simulink model "compare"  (R2024b)
settings: Solver=FixedStepAuto  StartTime=0.0  StopTime=200  FixedStep=1/fs  RelTol=1e-3
values from neighbouring files (symbols this model uses):
  s = 1i * omega_full    [find_best_kc.m]
libraries: simulink_extras x4, dspfdesign x2, slctrl_linear x1, cstblocks x1, slctrl_fre x1
settings Model: Creator=caohuaqi  LastModifiedBy=Caohuaqi

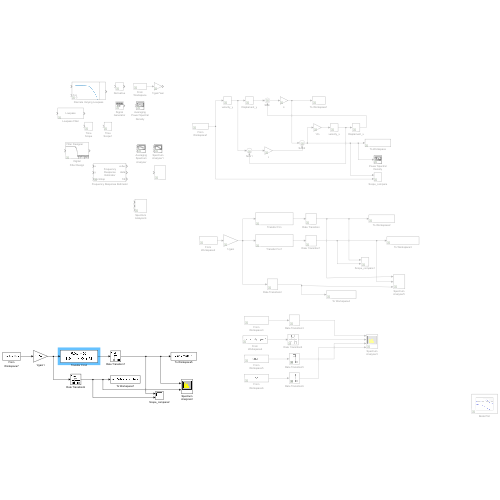
[thumbnail: Simulink's stored preview of the top-level diagram]
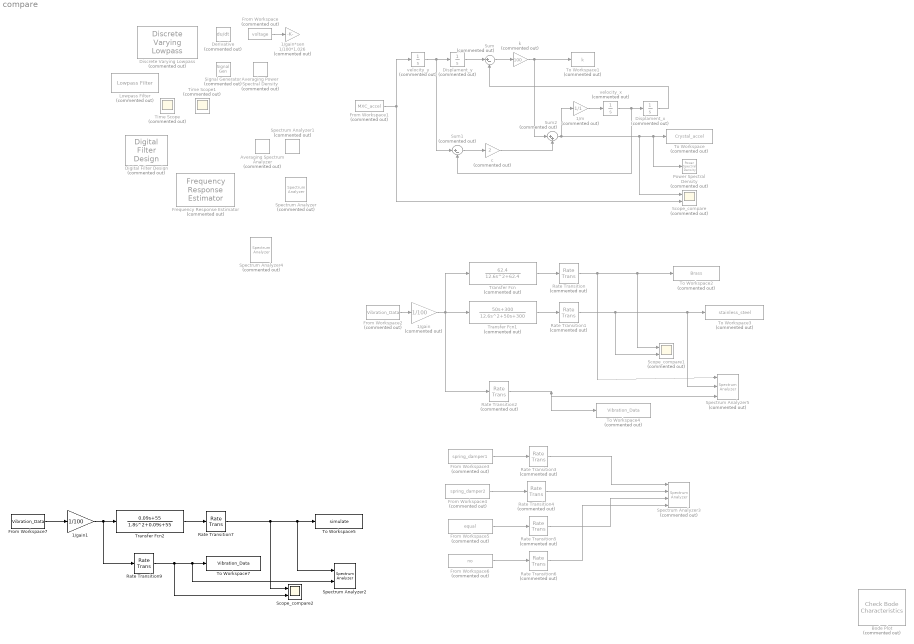
== system compare ==
  1/gain : Gain  Commented=on  Gain=1/100
  1/gain*sen : Gain  Commented=on  Gain=1/100*1.026
  1/gain1 : Gain  Gain=1/100
  1/m : Gain  Commented=on  Gain=1/1
  Averaging Power Spectral Density : simulink_extras/Additional Sinks/Averaging Power Spectral Density  Commented=on  npts=128  fftpts=512  HowOften=64  sampleT=0.1
  Averaging Spectrum Analyzer : simulink_extras/Additional Sinks/Averaging Spectrum Analyzer  Commented=on  npts=256  fftpts=256  HowOften=64  sampleT=0.1
  Bode Plot : slctrl_linear/Check Bode  Characteristics  Commented=on  InstantiateOnLoad=on  SaveOperatingPoints=off  LinearizationIOs={}  LinearizeAt=SnapshotTimes  SnapshotTimes=[0]  TriggerType=rising  SampleTime=auto  RateConversionMethod=zoh  PreWarpFreq=10  UseExactDelayModel=off  UseFullBlockNameLabels=off  UseBusSignalLabels=off  enabled=on  stopWhenAssertionFail=off  export=off  ViewDlgPos=[]  OpenViewOnLoad=off  LaunchViewOnOpen=off  FrequencyUnits=rad/s  MagnitudeUnits=dB  PhaseUnits=deg  TimeUnits=seconds  EnableUpperBound=off  UpperBoundFrequencies=[]  UpperBoundMagnitudes=[]  EnableLowerBound=off  LowerBoundFrequencies=[]  LowerBoundMagnitudes=[]
      settings: LibrarySourceBlock=slctrlblks/Linear Analysis Plots/Bode Plot  SaveToWorkspace=off  SaveName=sys
  Derivative : Derivative  Commented=on
  Digital Filter Design : dspfdesign/Digital Filter Design  Commented=on  mwdsp_browser_bugfix_var=off
  Discrete Varying Lowpass : cstblocks/Linear Parameter Varying/Discrete Varying Lowpass  Commented=on  N=1  w0=0  Ts=1
  Displament_x : Integrator  Commented=on
  Displament_y : Integrator  Commented=on
  Frequency Response Estimator : slctrl_fre/Frequency Response Estimator  Commented=on  DiscreteTs=0.1  OutputMode=control action + perturbation  BlockDataType=double  SineSource=Block parameters  Frequencies=[0.5 1 2]  FreqUnits=rad/s  Amplitudes=1  NumOfFreq=3  ExperimentMode=Sinestream  NumOfSetPeriod=2  NumOfEstPeriod=4  NumOfSlowestPeriod=3  NumOfPRBSPeriod=1  UseAutogenNumOfPRBSPeriod=off  PRBSSignalOrder=12  UseAutogenPRBSSignalOrder=off  EstimationMode=Online  UseBodePlot=off  BaselinePlant=[]  PlotRefreshFactor=100  UseExternalTs=off  BodePlotChoice=VariantNull  ExperimentChoice=VariantSS  OutputChoice=VariantCandD  CompiledTsChoice=InternalTs
      settings: LibrarySourceBlock=slctrlblks/Frequency Response Estimation/Frequency Response Estimator
  From Workspace : FromWorkspace  Commented=on  VariableName=voltage
  From Workspace1 : FromWorkspace  Commented=on  VariableName=MXC_accel
  From Workspace2 : FromWorkspace  Commented=on  VariableName=Vibration_Data
  From Workspace3 : FromWorkspace  Commented=on  VariableName=spring_damper1
  From Workspace4 : FromWorkspace  Commented=on  VariableName=spring_damper2
  From Workspace5 : FromWorkspace  Commented=on  VariableName=equal
  From Workspace6 : FromWorkspace  Commented=on  VariableName=no
  From Workspace7 : FromWorkspace  VariableName=Vibration_Data
  Lowpass Filter : dspfdesign/Lowpass Filter  Commented=on  FilterType=FIR  DesignForMinimumOrder=on  FilterOrder=50  PassbandFrequency=0.3628  StopbandFrequency=0.5442  PassbandRipple=0.1  StopbandAttenuation=80  SampleRateMode=Use normalized frequency (0 to 1)  SampleRate=44100  SimulateUsing=Interpreted execution  roundingMode=Floor  coeffsDataTypeStr=fixdt(1,16)
  Power Spectral Density : simulink_extras/Additional Sinks/Power Spectral Density  Commented=on  npts=128  fftpts=512  HowOften=64  sampleT=0.1
  Rate Transition{,1..6} (7 alike) : RateTransition  Commented=on  OutPortSampleTimeOpt=Inherit
  Rate Transition7 : RateTransition  OutPortSampleTimeOpt=Inherit
  Rate Transition9 : RateTransition  OutPortSampleTimeOpt=Inherit
  Scope_compare : Scope  Commented=on  NumInputPorts=2
  Scope_compare1 : Scope  Commented=on  NumInputPorts=2
  Scope_compare2 : Scope  NumInputPorts=2
  Signal Generator : SignalGenerator  Commented=on  Frequency=10
  Spectrum Analyzer : SpectrumAnalyzer  Commented=on  Method=Welch  PlotAsTwoSidedSpectrum=off  AveragingMethod=Exponential
  Spectrum Analyzer1 : simulink_extras/Additional Sinks/Spectrum Analyzer  Commented=on  npts=256  fftpts=256  HowOften=64  sampleT=0.1
  Spectrum Analyzer2 : SpectrumAnalyzer  NumInputPorts=2  WindowPosition=[801.000000,144.000000,1094.000000,562.000000,]  ScopeFrameLocation=window  SpectrumType=Power density  Method=Welch  PlotAsTwoSidedSpectrum=off  FrequencyScale=Log  FrequencyResolutionMethod=Window length  WindowLength=100000  FFTLengthSource=Property  FFTLength=100000  StartFrequency=0.01  StopFrequency=100  OverlapPercent=50  SpectrumUnits=dBm/Hz  YLimits=[-280.35527972,7.89698847]  ShowLegend=on
  Spectrum Analyzer3 : SpectrumAnalyzer  Commented=on  NumInputPorts=4  WindowPosition=[586.000000,265.000000,800.000000,500.000000,]  ScopeFrameLocation=window  SpectrumType=Power density  Method=Welch  PlotAsTwoSidedSpectrum=off  FrequencyScale=Log  FrequencySpan=Start and stop frequencies  StartFrequency=0.01  StopFrequency=100  AveragingMethod=Exponential  SpectrumUnits=dBm/Hz  YLimits=[-160.54617526,-4.99328965]  ShowLegend=on  SelectedToolstripTab=spectrumAnalyzerToolstrip.measurementsTab  MeasurementChannel=2
  Spectrum Analyzer4 : SpectrumAnalyzer  Commented=on  NumInputPorts=3  WindowPosition=[586.000000,265.000000,800.000000,500.000000,]  ScopeFrameLocation=window  SpectrumType=Power density  Method=Welch  PlotAsTwoSidedSpectrum=off  FrequencyScale=Log  FrequencySpan=Start and stop frequencies  StartFrequency=0.01  StopFrequency=100  AveragingMethod=Exponential  SpectrumUnits=dBm/Hz  YLimits=[-139.50728171,-33.44298748]  ShowLegend=on  SelectedToolstripTab=spectrumAnalyzerToolstrip.estimationTab  MeasurementChannel=2
  Spectrum Analyzer5 : SpectrumAnalyzer  Commented=on  NumInputPorts=3  WindowPosition=[1099.000000,643.000000,1094.000000,562.000000,]  ScopeFrameLocation=window  SpectrumType=Power density  Method=Welch  PlotAsTwoSidedSpectrum=off  FrequencyScale=Log  FrequencyResolutionMethod=Window length  WindowLength=100000  FFTLengthSource=Property  FFTLength=100000  StartFrequency=0.01  StopFrequency=100  OverlapPercent=50  SpectrumUnits=dBm/Hz  YLimits=[-254.98471041500628,63.29016997740334]  ShowLegend=on  SelectedToolstripTab=spectrumAnalyzerToolstrip.channelMeasurementsTab
  Sum : Sum  Commented=on  Inputs=|+-
  Sum1 : Sum  Commented=on  Inputs=|+-
  Sum2 : Sum  Commented=on  Inputs=|++
  Time Scope : Scope  Commented=on
  Time Scope1 : Scope  Commented=on
  To Workspace : ToWorkspace  Commented=on  VariableName=Crystal_accel  SaveFormat=Timeseries  SampleTime=-1
  To Workspace1 : ToWorkspace  Commented=on  VariableName=k  SaveFormat=Structure With Time  SampleTime=-1
  To Workspace2 : ToWorkspace  Commented=on  VariableName=Brass  SaveFormat=Timeseries  SampleTime=-1
  To Workspace3 : ToWorkspace  Commented=on  VariableName=stainless_steel  SaveFormat=Timeseries  SampleTime=-1
  To Workspace4 : ToWorkspace  Commented=on  VariableName=Vibration_Data  SaveFormat=Timeseries  SampleTime=-1
  To Workspace5 : ToWorkspace  VariableName=simulate  SaveFormat=Timeseries  SampleTime=-1
  To Workspace7 : ToWorkspace  VariableName=Vibration_Data  SaveFormat=Timeseries  SampleTime=-1
  Transfer Fcn : TransferFcn  Commented=on  Numerator=[0 62.4]  Denominator=[12.6 0 62.4]
  Transfer Fcn1 : TransferFcn  Commented=on  Numerator=[50 300]  Denominator=[12.6 50 300]
  Transfer Fcn2 : TransferFcn  Numerator=[0.09 55]  Denominator=[1.8 0.09 55]
  c : Gain  Commented=on  Gain=2
  k : Gain  Commented=on  Gain=100
  velocity_x : Integrator  Commented=on
  velocity_y : Integrator  Commented=on
  wires:
  velocity_y/1 -> Sum1/1, Displament_y/1
  Sum/1 -> k/1
  Sum1/1 -> c/1
  k/1 -> To Workspace1/1, Sum2/1
  c/1 -> Sum2/2
  Sum2/1 -> Scope_compare/1, Power Spectral Density/1, To Workspace/1, 1/m/1
  1/m/1 -> velocity_x/1
  velocity_x/1 -> Displament_x/1, Sum1/2
  Displament_x/1 -> Sum/2
  Displament_y/1 -> Sum/1
  From Workspace/1 -> 1/gain*sen/1
  From Workspace1/1 -> Scope_compare/2, velocity_y/1
  Transfer Fcn/1 -> Rate Transition/1
  Transfer Fcn1/1 -> Rate Transition1/1
  Rate Transition/1 -> Spectrum Analyzer5/1, To Workspace2/1, Scope_compare1/1
  Rate Transition1/1 -> To Workspace3/1, Spectrum Analyzer5/2, Scope_compare1/2
  Rate Transition2/1 -> Spectrum Analyzer5/3, To Workspace4/1
  From Workspace6/1 -> Rate Transition6/1
  From Workspace5/1 -> Rate Transition5/1
  From Workspace4/1 -> Rate Transition4/1
  From Workspace3/1 -> Rate Transition3/1
  Rate Transition3/1 -> Spectrum Analyzer3/1
  Rate Transition4/1 -> Spectrum Analyzer3/2
  Rate Transition5/1 -> Spectrum Analyzer3/3
  Rate Transition6/1 -> Spectrum Analyzer3/4
  From Workspace2/1 -> 1/gain/1
  1/gain/1 -> Transfer Fcn/1, Rate Transition2/1, Transfer Fcn1/1
  Rate Transition7/1 -> Spectrum Analyzer2/1, To Workspace5/1, Scope_compare2/1
  Rate Transition9/1 -> Scope_compare2/2, Spectrum Analyzer2/2, To Workspace7/1
  Transfer Fcn2/1 -> Rate Transition7/1
  1/gain1/1 -> Rate Transition9/1, Transfer Fcn2/1
  From Workspace7/1 -> 1/gain1/1
